simulink model "linear_shift_feedback_register_demo"  (R2022b)
settings: Solver=VariableStepAuto  StartTime=0.0  StopTime=200  RelTol=1e-3
libraries: commseqgen3 x2
settings Model: Creator=Jason.McGinthy  LastModifiedBy=Jason.McGinthy

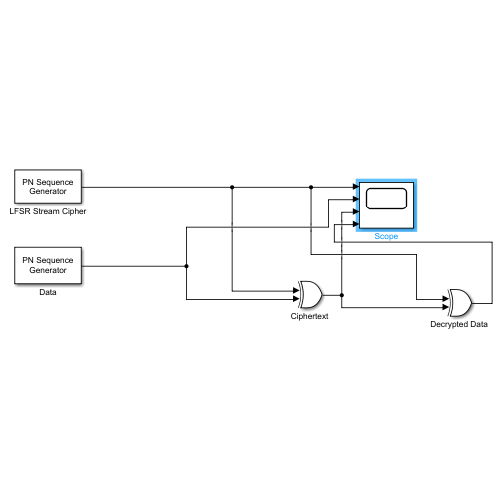
[thumbnail: Simulink's stored preview of the top-level diagram]
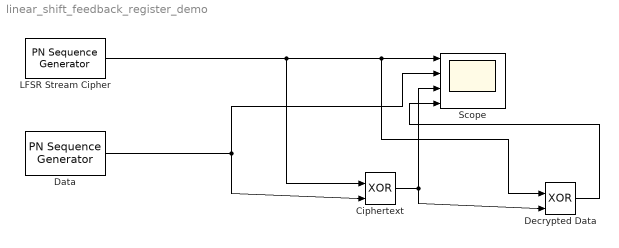
== system linear_shift_feedback_register_demo ==
  Ciphertext : Logic  Operator=XOR  IconShape=distinctive  AllPortsSameDT=off  OutDataTypeStr=boolean
  Data : commseqgen3/PN Sequence Generator  poly=[53 52 51 47 0]  ini_sta=randi([0 1], 1, 53)  outBitMaskSource=Dialog parameter  shift=1  outVarSiz=off  maxOutSizeMode=Dialog parameter  maxOutSize=[8 1]  Ts=1  sampPerFrame=1  reset=off  bitPackedOutputs=off  outDataType=double  numPackedBits=8  bitPackDataSigned=off  bitPackedOutDType=Smallest integer
      settings: LibrarySourceBlock=|
      | commhdlsource/PN Sequence
      | Generator
  Decrypted Data : Logic  Operator=XOR  IconShape=distinctive  AllPortsSameDT=off  OutDataTypeStr=boolean
  LFSR Stream Cipher : commseqgen3/PN Sequence Generator  poly=[53 52 51 47 0]  ini_sta=randi([0 1],1, 53)  outBitMaskSource=Dialog parameter  shift=1  outVarSiz=off  maxOutSizeMode=Dialog parameter  maxOutSize=[8 1]  Ts=1  sampPerFrame=1  reset=off  bitPackedOutputs=off  outDataType=double  numPackedBits=8  bitPackDataSigned=off  bitPackedOutDType=Smallest integer
      settings: LibrarySourceBlock=|
      | commhdlsource/PN Sequence
      | Generator
  Scope : Scope  NumInputPorts=4
  wires:
  LFSR Stream Cipher/1 -> Ciphertext/1, Decrypted Data/1, Scope/1
  Data/1 -> Ciphertext/2, Scope/2
  Ciphertext/1 -> Decrypted Data/2, Scope/3
  Decrypted Data/1 -> Scope/4
